simulink model "SIM_SAD_DEMO"  (R2025b)
settings: Solver=ode5  StartTime=0.0  StopTime=T/10  FixedStep=0.1  RelTol=1e-3
model workspace (MAT data in the model file):
  Pnull = Simulink.Parameter
  Pnull.Value = Simulink.data.Expression
  Pnull.Value.ExpressionString = "zeros(3,1)"
  Pnull.Complexity = 'real'
  Pnull.Dimensions = -1
  Pnull.DataType = 'auto'
  rho_albedo_medio = Simulink.Parameter
  rho_albedo_medio.Value = 0.3
  rho_albedo_medio.Complexity = 'real'
  rho_albedo_medio.Dimensions = [1 1]
  rho_albedo_medio.DataType = 'auto'
values from neighbouring files (symbols this model uses):
  Aree = zeros(10,1)    [SCRIPT_SAD_DEMO.m]    (also in lab_7.m)
  c = astroConstants(5)*1e3    [SCRIPT_SAD_DEMO.m]    (also in lab_7.m)
  draan = 1.99096871e-7    (= 1.99096871e-07)    [SCRIPT_SAD_DEMO.m]
  eps_E = deg2rad(astroConstants(63))    [SCRIPT_SAD_DEMO.m]    (also in lab_7.m)
  F_e = 1358    [SCRIPT_SAD_DEMO.m]    (also in lab_7.m)
  j_B = [0.01; 0.05; 0.01]    [SCRIPT_SAD_DEMO.m]    (also in lab_7.m)
  J_depl = [100.9, 0, 0;           0, 25.1, 0;           0, 0, 91.6]*1e-2    [SCRIPT_SAD_DEMO.m]    (also in lab_7.m)
  JD0 = juliandate(startTime)    [SCRIPT_SAD_DEMO.m]
  kep = [a,e,incl,raan,w,theta]    [SCRIPT_SAD_DEMO.m]    (also in lab_7.m)
  mu = astroConstants(13)    [SCRIPT_SAD_DEMO.m]    (also in lab_7.m)
  n = sqrt( (mu/ (a)^3))    [SCRIPT_SAD_DEMO.m]    (also in lab_7.m = sqrt((mu/ ((a/1000)^3))))
  n_sun = 2*pi/T_sun    (= 1.99238499086e-07)    [SCRIPT_SAD_DEMO.m]    (also in lab_7.m)
  Nmat = [ ... (first row only)    [SCRIPT_SAD_DEMO.m]    (also in lab_7.m)
  r_sun = 1*AU    [SCRIPT_SAD_DEMO.m]    (also in lab_7.m = 1*ua)
  Re = astroConstants(23)    [SCRIPT_SAD_DEMO.m]    (also in lab_7.m)
  rf = [ ... (first row only)    [SCRIPT_SAD_DEMO.m]    (also in lab_7.m)
  rhod = 0.1*ones(10,1)    [SCRIPT_SAD_DEMO.m]    (also in lab_7.m)
  rhos = zeros(10,1)    [SCRIPT_SAD_DEMO.m]    (also in lab_7.m)
  theta = 0    [SCRIPT_SAD_DEMO.m]    (also in lab_7.m)
undefined symbols (not defined in the file or in its folder): avec, bvec, DiscIntNeverNeededParam, dspblkCoreblockFVToolHelper, gcbh, Gyro, Magmeter, q, SRP, Sun_sensor
libraries: LIBRARY_SAD x37, matrix_library x28
(part 1 of 3)
settings Model: Creator=fabio  LastModifiedBy=delil

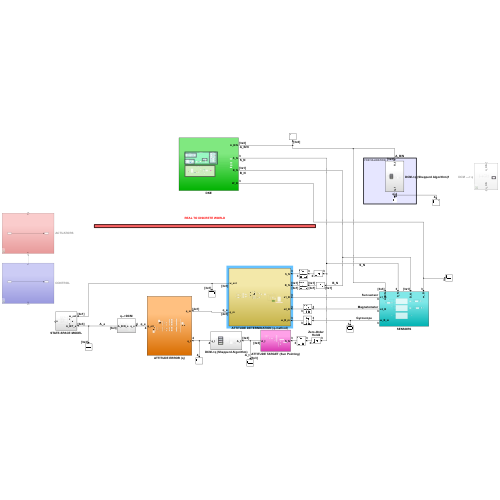
[thumbnail: Simulink's stored preview of the top-level diagram]
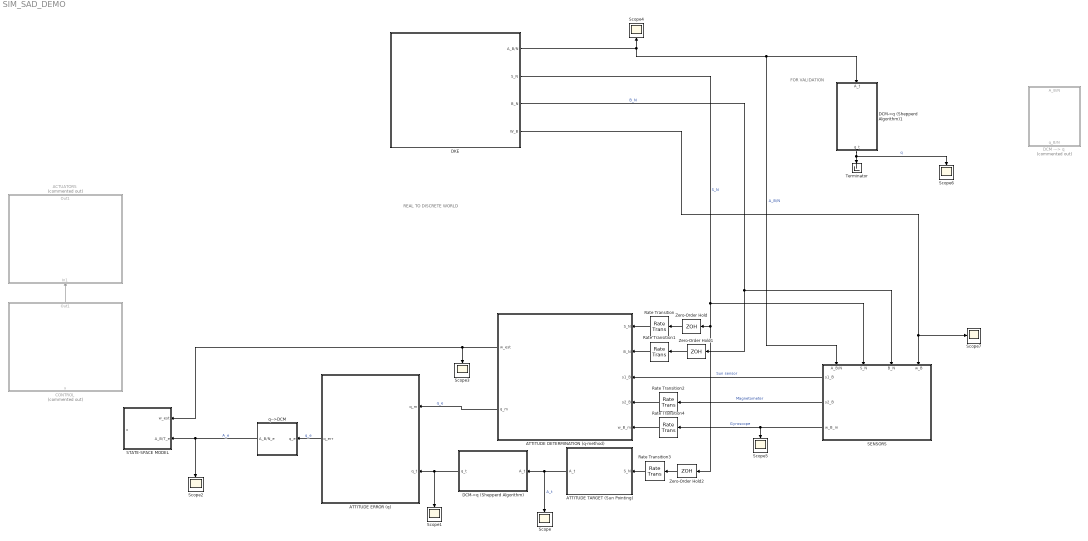
== system SIM_SAD_DEMO ==
  note: FOR VALIDATION
  note: REAL TO DISCRETE WORLD
  ACTUATORS : Subsystem  Commented=on
  ATTITUDE DETERMINATION (q-method) : Subsystem
  ATTITUDE ERROR (q) : Subsystem
  ATTITUDE TARGET (Sun Pointing) : Subsystem
  CONTROL : Subsystem  Commented=on
  DCM ---> q : Subsystem  Commented=on
  DCM->q (Shepperd Algorithm) : Subsystem
  DCM->q (Shepperd Algorithm)1 : Subsystem
  DKE : Subsystem
  Rate Transition{,1..4} (5 alike) : RateTransition  OutPortSampleTime=max(Sun_sensor.Ts,Magmeter.Ts)
  SENSORS : Subsystem
      settings: PortSchema="{\"entries\":[{\"content\":{\"sides\":[{\"content\":{\"connectorIds\":[\"In1\",\"In2\",\"In3\",\"In4\"]},\"type\":\"ConnectorPlacement.EquallySpacedRectSide\",\"uuid\":\"40962b30-3bcb-49e0-bc68-6aa3a31cfc97\"},{\"content\":{\"side\":\"RIGHT\"},\"type\":\"ConnectorPlacement.EquallySpacedRectSide\",\"uuid\":\"a8221d80-3d13-495d-884e-34f2ccc75f25\"},{\"content\":{\"connectorIds\":[\"Out1\",\"Out2\",\"Out3\"],\"side\":\"TOP\"},\"type\":\"ConnectorPlacement.EquallySpacedRectSide\",\"uuid\":\"62b0f620-b15f-4d6a-bcfa-939a48d36217\"}]},\"type\":\"ConnectorPlacement.EquallySpacedConnector\",\"uuid\":\"bc93d320-282b-4258-8528-17688a47c52b\"}],\"packageUris\":[\"http://schema.mathworks.com/mf0/Connector/R2020b\"],\"version\":\"1.0\"}"
  STATE-SPACE MODEL : Subsystem
  Scope{,1..7} (8 alike) : Scope
      Scope settings: ActiveDisplayYMinimum=-1  ActiveDisplayYMaximum=1  DataLoggingVariableName=ScopeData55
      Scope1 settings: ActiveDisplayYMinimum=-1  ActiveDisplayYMaximum=1  DataLoggingVariableName=ScopeData81
      Scope2 settings: ActiveDisplayYMinimum=-1.2400140928314325  ActiveDisplayYMaximum=1.248890454759048  DataLoggingVariableName=ScopeData60
      Scope3 settings: ActiveDisplayYMinimum=-0.92000036614875291  ActiveDisplayYMaximum=5.28182468939155  DataLoggingVariableName=ScopeData72
      Scope4 settings: ActiveDisplayYMinimum=-1.2499999997091158  ActiveDisplayYMaximum=1.2499999999676794  DataLoggingVariableName=ScopeData71
      Scope5 settings: ActiveDisplayYMinimum=-0.010336393980870042  ActiveDisplayYMaximum=0.027780099120889055  DataLoggingVariableName=ScopeData83
      Scope6 settings: ActiveDisplayYMinimum=-1  ActiveDisplayYMaximum=1  DataLoggingVariableName=ScopeData82
      Scope7 settings: ActiveDisplayYMinimum=-0.018485878503427311  ActiveDisplayYMaximum=0.018741294883568061  DataLoggingVariableName=ScopeData84
  Terminator : Terminator
  Zero-Order Hold : ZeroOrderHold  SampleTime=max(Sun_sensor.Ts,Magmeter.Ts)
  Zero-Order Hold1 : ZeroOrderHold  SampleTime=max(Sun_sensor.Ts,Magmeter.Ts)
  Zero-Order Hold2 : ZeroOrderHold  SampleTime=max(Sun_sensor.Ts,Magmeter.Ts)
  q-->DCM : Subsystem
  wires:
  DCM->q (Shepperd Algorithm)1/1(q_t) -> Scope6/1, Terminator/1  "q"
  SENSORS/2(s2_B) -> Rate Transition2/1  "Magnetometer"
  ATTITUDE TARGET (Sun Pointing)/1(A_t) -> Scope/1, DCM->q (Shepperd Algorithm)/1(A_t)  "A_t"
  DCM->q (Shepperd Algorithm)/1(q_t) -> Scope1/1, ATTITUDE ERROR (q)/2(q_t)
  q-->DCM/1(A_B/N_e) -> Scope2/1, STATE-SPACE MODEL/2(A_B/T_e)  "A_e"
  ATTITUDE ERROR (q)/1(q_err) -> q-->DCM/1(q_e)  "q_e"
  Zero-Order Hold/1 -> Rate Transition/1
  Rate Transition/1 -> ATTITUDE DETERMINATION (q-method)/1(S_N)
  Zero-Order Hold1/1 -> Rate Transition1/1
  Rate Transition1/1 -> ATTITUDE DETERMINATION (q-method)/2(B_N)
  Zero-Order Hold2/1 -> Rate Transition3/1
  Rate Transition3/1 -> ATTITUDE TARGET (Sun Pointing)/1(S_N)
  CONTROL/1(Out1) -> ACTUATORS/1(In1)
  DKE/4(W_B) -> SENSORS/4(w_B), Scope7/1
  SENSORS/3(w_B_m) -> Scope5/1, Rate Transition4/1  "Gyroscope"
  ATTITUDE DETERMINATION (q-method)/2(q_m) -> ATTITUDE ERROR (q)/1(q_m)  "q_e"
  Rate Transition2/1 -> ATTITUDE DETERMINATION (q-method)/4(s2_B)
  ATTITUDE DETERMINATION (q-method)/1(w_est) -> Scope3/1, STATE-SPACE MODEL/1(w_est)
  DKE/3(B_N) -> SENSORS/3("B_N "), Zero-Order Hold1/1  "B_N"
  SENSORS/1(s1_B) -> ATTITUDE DETERMINATION (q-method)/3(s1_B)  "Sun sensor"
  DKE/2(S_N) -> SENSORS/2(S_N), Zero-Order Hold/1, Zero-Order Hold2/1  "S_N"
  DKE/1(A_B/N) -> Scope4/1, DCM->q (Shepperd Algorithm)1/1(A_t), SENSORS/1(A_B/N)  "A_B/N"
  Rate Transition4/1 -> ATTITUDE DETERMINATION (q-method)/5(w_B_m)

== system SIM_SAD_DEMO/ACTUATORS ==
  In1 : Inport
  Out1 : Outport
  wires:
  In1/1 -> Out1/1

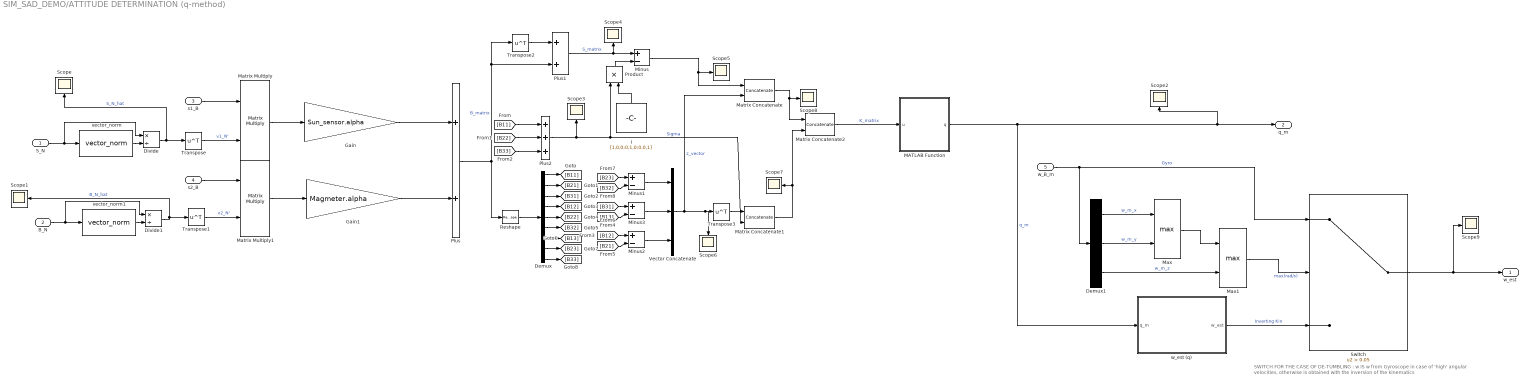
== system SIM_SAD_DEMO/ATTITUDE DETERMINATION (q-method) ==
  note: SWITCH FOR THE CASE OF DE-TUMBLING : w IS w from Gyroscope in case of 'high' angular velocities, otherwise is obtained with the inversion of the kinematics
  S_N : Inport
  B_N : Inport  Port=2
  s1_B : Inport  Port=3
  s2_B : Inport  Port=4
  w_B_m : Inport  Port=5
  Demux : Demux  Outputs=9
  Demux1 : Demux  Outputs=3
  Divide : Product  Inputs=*/
  Divide1 : Product  Inputs=*/
  Gain : Gain  Gain=Sun_sensor.alpha
  Gain1 : Gain  Gain=Magmeter.alpha
  I : Constant  Value=[1,0,0;0,1,0;0,0,1]
  MATLAB Function : MATLAB Function  TreatAsAtomicUnit=on  SystemSampleTime=q.Ts
  Matrix Concatenate : Concatenate  Mode=Multidimensional array  ConcatenateDimension=2
  Matrix Concatenate1 : Concatenate  Mode=Multidimensional array  ConcatenateDimension=2
  Matrix Concatenate2 : Concatenate  Mode=Multidimensional array
  Matrix Multiply : Product  Multiplication=Matrix(*)
  Matrix Multiply1 : Product  Multiplication=Matrix(*)
  Max : MinMax  Function=max  Inputs=2
  Max1 : MinMax  Function=max  Inputs=2
  Minus{,1..3} (4 alike) : Sum  Inputs=+-
  Plus : Sum
  Plus1 : Sum
  Plus2 : Sum  Inputs=+++
  Product : Product
  Reshape : Reshape  OutputDimensionality=Customize  OutputDimensions=[9,1]
  Scope{,1..9} (10 alike) : Scope
      Scope settings: ActiveDisplayYMinimum=-0.12499999999999997  ActiveDisplayYMaximum=1.125  DataLoggingVariableName=ScopeData61
      Scope1 settings: ActiveDisplayYMinimum=-0.60786913937993192  ActiveDisplayYMaximum=1.0990417923572595  DataLoggingVariableName=ScopeData62
      Scope2 settings: ActiveDisplayYMinimum=-0.9533532616313245  ActiveDisplayYMaximum=1.1062124291352333  DataLoggingVariableName=ScopeData74
      Scope3 settings: ActiveDisplayYMinimum=-1  ActiveDisplayYMaximum=1  DataLoggingVariableName=ScopeData75
      Scope4 settings: DataLoggingVariableName=ScopeData76
      Scope5 settings: ActiveDisplayYMinimum=-1  ActiveDisplayYMaximum=1  DataLoggingVariableName=ScopeData77
      Scope6 settings: DataLoggingVariableName=ScopeData78
      Scope7 settings: ActiveDisplayYMinimum=-1  ActiveDisplayYMaximum=1  DataLoggingVariableName=ScopeData79
      Scope8 settings: ActiveDisplayYMinimum=-1.2343387282561236  ActiveDisplayYMaximum=1.1812725103052406  DataLoggingVariableName=ScopeData80
      Scope9 settings: ActiveDisplayYMinimum=-0.28605679058813616  ActiveDisplayYMaximum=0.3787347965228936  DataLoggingVariableName=ScopeData85
  Switch : Switch  Criteria=u2 > Threshold  Threshold=0.05  SaturateOnIntegerOverflow=off  InputSameDT=off
  Transpose{,1..3} (4 alike) : Math  Operator=transpose
  Vector Concatenate : Concatenate  NumInputs=3
  vector_norm : LIBRARY_SAD/vector_norm  SystemSampleTime=-1  VariantActivationTime=update diagram  EmptyChoice=off  PassThrough=off  PassThroughVariantControl=(default)  EmptyChoiceVariantControl=(default)  AllowFlexibleInterface=on  Latency=0  AutoFrameSizeCalculation=off
  vector_norm1 : LIBRARY_SAD/vector_norm  SystemSampleTime=-1  VariantActivationTime=update diagram  EmptyChoice=off  PassThrough=off  PassThroughVariantControl=(default)  EmptyChoiceVariantControl=(default)  AllowFlexibleInterface=on  Latency=0  AutoFrameSizeCalculation=off
  w_est (q) : Subsystem
  w_est : Outport
  q_m : Outport  Port=2
  wires:
  vector_norm/1 -> Divide/2
  Demux/6 -> [B32]
  Divide/1 -> Scope/1, Transpose/1  "S_N_hat"
  Gain/1 -> Plus/1
  [B32] -> Minus1/2
  Gain1/1 -> Plus/2
  S_N/1 -> Divide/1, vector_norm/1
  Plus2/1 -> Scope3/1, Product/1, Matrix Concatenate1/2  "Sigma"
  B_N/1 -> Divide1/1, vector_norm1/1
  Demux/4 -> [B12]
  Plus/1 -> Reshape/1, Transpose2/1, Plus1/2  "B_matrix"
  Divide1/1 -> Scope1/1, Transpose1/1  "B_N_hat"
  [B12] -> Minus2/1
  Demux/3 -> [B31]
  Demux/8 -> [B23]
  Vector Concatenate/1 -> Matrix Concatenate/2, Transpose3/1, Scope6/1  "z_vector"
  Minus1/1 -> Vector Concatenate/1
  Minus2/1 -> Vector Concatenate/3
  Transpose2/1 -> Plus1/1
  [B11] -> Plus2/1
  Transpose/1 -> Matrix Multiply/2  "v1_N'"
  Minus/1 -> Scope5/1, Matrix Concatenate/1
  Matrix Concatenate1/1 -> Scope7/1, Matrix Concatenate2/2
  Demux/1 -> [B11]
  [B22] -> Plus2/2
  Matrix Multiply1/1 -> Gain1/1
  Demux/2 -> [B21]
  [B23] -> Minus1/1
  Demux/5 -> [B22]
  Matrix Multiply/1 -> Gain/1
  Demux/9 -> [B33]
  Reshape/1 -> Demux/1
  Demux/7 -> [B13]
  vector_norm1/1 -> Divide1/2
  [B33] -> Plus2/3
  Matrix Concatenate/1 -> Matrix Concatenate2/1, Scope8/1
  Transpose1/1 -> Matrix Multiply1/2  "v2_N'"
  Transpose3/1 -> Matrix Concatenate1/1
  Minus3/1 -> Vector Concatenate/2
  [B31] -> Minus3/1
  Plus1/1 -> Minus/1, Scope4/1  "S_matrix"
  [B13] -> Minus3/2
  [B21] -> Minus2/2
  Product/1 -> Minus/2
  I/1 -> Product/2
  s1_B/1 -> Matrix Multiply/1
  s2_B/1 -> Matrix Multiply1/1
  MATLAB Function/1(q) -> w_est (q)/1(q_m), q_m/1, Scope2/1  "q_m"
  Switch/1 -> Scope9/1, w_est/1
  Matrix Concatenate2/1 -> MATLAB Function/1(u)  "K_matrix"
  Max/1 -> Max1/1
  Demux1/3 -> Max1/2  "w_m_z"
  Demux1/2 -> Max/2  "w_m_y"
  Demux1/1 -> Max/1  "w_m_x"
  w_B_m/1 -> Switch/1, Demux1/1  "Gyro"
  Max1/1 -> Switch/2  "max(rad/s)"
  w_est (q)/1(w_est) -> Switch/3  "Inverting Kin"

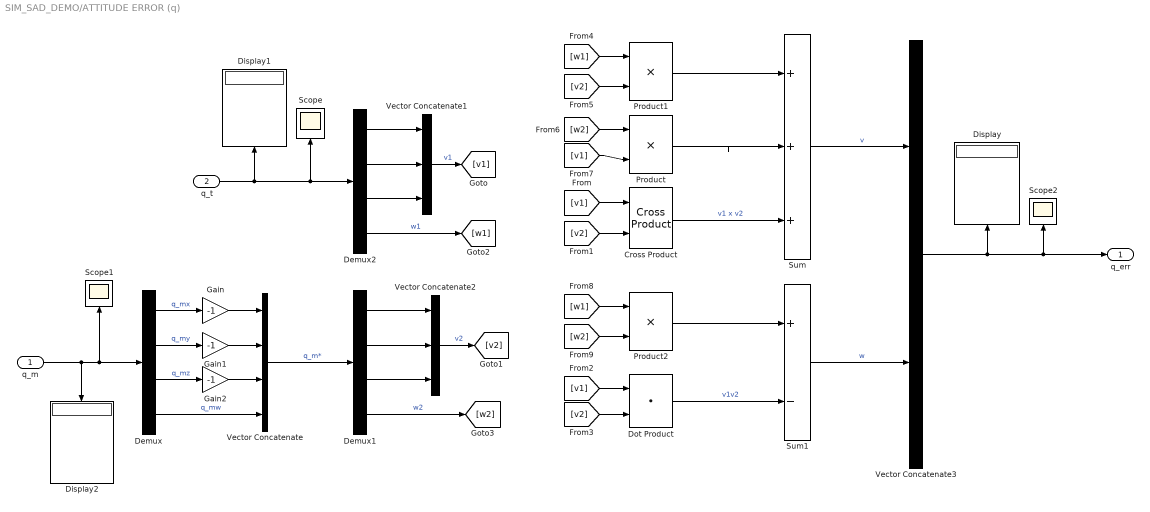
== system SIM_SAD_DEMO/ATTITUDE ERROR (q) ==
  q_m : Inport
  q_t : Inport  Port=2
  Cross Product : matrix_library/Cross Product
  Demux : Demux
  Demux1 : Demux
  Demux2 : Demux
  Display : Display
  Display1 : Display
  Display2 : Display
  Dot Product : DotProduct  OutDataTypeStr=Inherit: Inherit via internal rule
  Gain : Gain  Gain=-1
  Gain1 : Gain  Gain=-1
  Gain2 : Gain  Gain=-1
  Product : Product
  Product1 : Product
  Product2 : Product
  Scope : Scope
      settings: ActiveDisplayYMinimum=-0.12923710595911297  ActiveDisplayYMaximum=1.1085905151201327  DataLoggingVariableName=ScopeData63
  Scope1 : Scope
      settings: ActiveDisplayYMinimum=-1.1944830769885011  ActiveDisplayYMaximum=1.2235445279118087  DataLoggingVariableName=ScopeData64
  Scope2 : Scope
      settings: ActiveDisplayYMinimum=-1  ActiveDisplayYMaximum=1  DataLoggingVariableName=ScopeData65
  Sum : Sum  Inputs=+++
  Sum1 : Sum  Inputs=+-
  Vector Concatenate : Concatenate  NumInputs=4
  Vector Concatenate1 : Concatenate  NumInputs=3
  Vector Concatenate2 : Concatenate  NumInputs=3
  Vector Concatenate3 : Concatenate
  q_err : Outport
  wires:
  q_m/1 -> Scope1/1, Demux/1, Display2/1
  q_t/1 -> Demux2/1, Scope/1, Display1/1
  Demux/1 -> Gain/1  "q_mx"
  Demux/2 -> Gain1/1  "q_my"
  Demux/3 -> Gain2/1  "q_mz"
  Demux/4 -> Vector Concatenate/4  "q_mw"
  Gain2/1 -> Vector Concatenate/3
  Gain1/1 -> Vector Concatenate/2
  Gain/1 -> Vector Concatenate/1
  Vector Concatenate/1 -> Demux1/1  "q_m*"
  Demux1/1 -> Vector Concatenate2/1
  Demux1/2 -> Vector Concatenate2/2
  Demux1/3 -> Vector Concatenate2/3
  Demux1/4 -> [w2]  "w2"
  Demux2/1 -> Vector Concatenate1/1
  Demux2/2 -> Vector Concatenate1/2
  Demux2/3 -> Vector Concatenate1/3
  Vector Concatenate1/1 -> [v1]  "v1"
  Demux2/4 -> [w1]  "w1"
  Cross Product/1 -> Sum/3  "v1 x v2"
  Dot Product/1 -> Sum1/2  "v1v2"
  [v1] -> Cross Product/1
  Vector Concatenate2/1 -> [v2]  "v2"
  [v2] -> Cross Product/2
  [v1] -> Dot Product/1
  [v2] -> Dot Product/2
  [w1] -> Product1/1
  [v2] -> Product1/2
  [v1] -> Product/2
  [w2] -> Product/1
  Product1/1 -> Sum/1
  Product/1 -> Sum/2
  [w1] -> Product2/1
  [w2] -> Product2/2
  Product2/1 -> Sum1/1
  Sum/1 -> Vector Concatenate3/1  "v"
  Sum1/1 -> Vector Concatenate3/2  "w"
  Vector Concatenate3/1 -> Scope2/1, q_err/1, Display/1

== system SIM_SAD_DEMO/ATTITUDE TARGET (Sun Pointing) ==
  note: BORESIGHT AXIS : axis which points the Sun
  S_N : Inport
  Constant{1..2,4,6,8..11} (8 alike) : Constant  Value=0
  Constant{3,5,7,12} (4 alike) : Constant
  Cross Product : matrix_library/Cross Product
  Cross Product1 : matrix_library/Cross Product
  Display : Display
  Display1 : Display
  MatrixMultiply : Product  Multiplication=Matrix(*)
  Normalized Vector : Subsystem
  Normalized Vector2 : Subsystem
  Scope{,1..4} (5 alike) : Scope
      Scope settings: ActiveDisplayYMinimum=-1  ActiveDisplayYMaximum=1  DataLoggingVariableName=ScopeData62
      Scope1 settings: ActiveDisplayYMinimum=-1  ActiveDisplayYMaximum=1  DataLoggingVariableName=ScopeData66
      Scope2 settings: ActiveDisplayYMinimum=-1  ActiveDisplayYMaximum=1  DataLoggingVariableName=ScopeData69
      Scope3 settings: ActiveDisplayYMinimum=-1  ActiveDisplayYMaximum=1  DataLoggingVariableName=ScopeData70
      Scope4 settings: ActiveDisplayYMinimum=-1  ActiveDisplayYMaximum=1  DataLoggingVariableName=ScopeData73
  Sum : Sum  Inputs=|+-
  Transpose : Math  Operator=transpose
  Vector Concatenate : Concatenate  NumInputs=3  Mode=Multidimensional array  ConcatenateDimension=2
  Vector Concatenate{1..4} (4 alike) : Concatenate  NumInputs=3
  Vector Concatenate5 : Concatenate  NumInputs=3  Mode=Multidimensional array  ConcatenateDimension=2
  A_t : Outport
  wires:
  S_N/1 -> Normalized Vector2/1(r)
  Normalized Vector2/1(s2_B) -> Cross Product/2, Cross Product1/1, Scope/1, Vector Concatenate/1  "x_t_hat"
  Vector Concatenate1/1 -> Cross Product/1  "k_hat"
  Cross Product/1 -> Normalized Vector/1(In1)
  Normalized Vector/1(Out1) -> Scope1/1, Vector Concatenate/2, Cross Product1/2  "y_t_hat"
  Cross Product1/1 -> Scope2/1, Vector Concatenate/3  "z_t_hat"
  Vector Concatenate/1 -> Scope4/1, A_t/1, MatrixMultiply/2, Transpose/1, Display/1  "A_T/N"
  Transpose/1 -> MatrixMultiply/1
  MatrixMultiply/1 -> Sum/1
  Vector Concatenate5/1 -> Display1/1, Sum/2  "I_matrix"
  Sum/1 -> Scope3/1
  Constant2/1 -> Vector Concatenate1/2
  Constant1/1 -> Vector Concatenate1/1
  Constant3/1 -> Vector Concatenate1/3
  Constant6/1 -> Vector Concatenate2/3
  Constant4/1 -> Vector Concatenate2/1
  Constant5/1 -> Vector Concatenate2/2
  Constant8/1 -> Vector Concatenate3/2
  Constant7/1 -> Vector Concatenate3/1
  Constant9/1 -> Vector Concatenate3/3
  Constant11/1 -> Vector Concatenate4/2
  Constant10/1 -> Vector Concatenate4/1
  Constant12/1 -> Vector Concatenate4/3
  Vector Concatenate3/1 -> Vector Concatenate5/1
  Vector Concatenate2/1 -> Vector Concatenate5/2
  Vector Concatenate4/1 -> Vector Concatenate5/3

== system SIM_SAD_DEMO/CONTROL ==
  x : Inport
  Out1 : Outport
  wires:
  x/1 -> Out1/1

== system SIM_SAD_DEMO/DCM ---> q ==
  note: CHECK BY RECONSTRUCTING A_B/N AND ORTHONORMALITY ERROR
  A_B/N : Inport
  Constant : Constant
  Demux : Demux  Outputs=9
  Divide{,1..3} (4 alike) : Product  Inputs=*/
  Gain : Gain  Gain=4
  Gain1 : Gain  Gain=4
  Gain2 : Gain  Gain=4
  Gain3 : Gain  Gain=1/2
  Reshape : Reshape  OutputDimensionality=Customize  OutputDimensions=[9,1]
  Sqrt : Sqrt
  Sum : Sum  Inputs=+-
  Sum1 : Sum  Inputs=++++
  Sum2 : Sum  Inputs=+-
  Sum3 : Sum  Inputs=+-
  Transpose1 : Math  Operator=transpose
  Vector Concatenate : Concatenate  NumInputs=4
  q-->DCM (CHECK) : Subsystem  Commented=on
  vector_norm : Subsystem
  q_B/N : Outport
  wires:
  A_B/N/1 -> Transpose1/1  "A_B/N"
  Transpose1/1 -> Reshape/1
  Divide3/1 -> q_B/N/1, q-->DCM (CHECK)/1(q_norm)  "q_norm"
  vector_norm/1(r_norm) -> Divide3/2
  Gain3/1 -> Vector Concatenate/4, Gain/1, Gain2/1, Gain1/1  "q4"
  Sqrt/1 -> Gain3/1
  Vector Concatenate/1 -> vector_norm/1(r), Divide3/1  "q"
  Gain2/1 -> Divide2/2
  Sum3/1 -> Divide2/1
  Gain1/1 -> Divide1/2
  Sum2/1 -> Divide1/1
  Gain/1 -> Divide/2
  Sum/1 -> Divide/1
  Constant/1 -> Sum1/1
  Sum1/1 -> Sqrt/1
  Divide2/1 -> Vector Concatenate/3  "q3"
  Divide1/1 -> Vector Concatenate/2  "q2"
  Divide/1 -> Vector Concatenate/1  "q1"
  Demux/9 -> Sum1/4  "A_33"
  Demux/8 -> Sum/2  "A_32"
  Demux/7 -> Sum2/1  "A_31"
  Demux/6 -> Sum/1  "A_23"
  Demux/5 -> Sum1/3  "A_22"
  Demux/4 -> Sum3/2  "A_21"
  Demux/3 -> Sum2/2  "A_13"
  Demux/2 -> Sum3/1  "A_12"
  Demux/1 -> Sum1/2  "A_11"
  Reshape/1 -> Demux/1

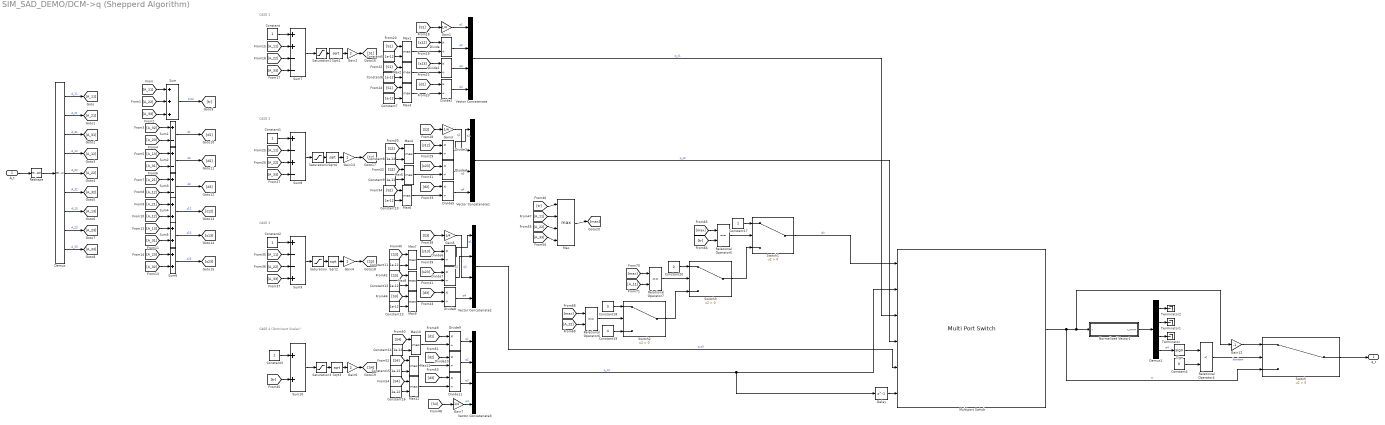
== system SIM_SAD_DEMO/DCM->q (Shepperd Algorithm) ==
  note: CASE 1
  note: CASE 2
  note: CASE 3
  note: CASE 4 (Dominant Scalar)
  A_t : Inport
  Constant{,1..3,17} (5 alike) : Constant
  Constant{5..16} (12 alike) : Constant  Value=1e-12
  Constant18 : Constant  Value=3
  Constant19 : Constant  Value=4
  Constant20 : Constant  Value=2
  Constant4 : Constant  Value=0
  Delay : Delay  DelayLength=1
  Demux : Demux  Outputs=9
  Demux1 : Demux
  Divide{,1..11} (12 alike) : Product  Inputs=*/
  Gain{1,3,5,7} (4 alike) : Gain  Gain=1/4
  Gain12 : Gain  Gain=-1
  Gain{2,4,6,13} (4 alike) : Gain  Gain=2
  Max : MinMax  Function=max  Inputs=4
  Max{1..12} (12 alike) : MinMax  Function=max  Inputs=2
  Multiport Switch : MultiPortSwitch  Inputs=4  DataPortForDefault=Additional data port  DiagnosticForDefault=Warning  SaturateOnIntegerOverflow=off
  Normalized Vector1 : Subsystem
  Relational Operator4 : RelationalOperator  Operator=<  OutDataTypeStr=boolean  RndMeth=Simplest  InputSameDT=off
  Relational Operator5 : RelationalOperator  Operator===  OutDataTypeStr=boolean  RndMeth=Simplest  InputSameDT=off
  Relational Operator6 : RelationalOperator  Operator===  OutDataTypeStr=boolean  RndMeth=Simplest  InputSameDT=off
  Relational Operator7 : RelationalOperator  Operator===  OutDataTypeStr=boolean  RndMeth=Simplest  InputSameDT=off
  Reshape : Reshape  OutputDimensionality=Customize  OutputDimensions=[9,1]
  Saturation{,1..3} (4 alike) : Saturate  UpperLimit=inf  LowerLimit=0
  Sign : Signum
  Sqrt{1..4} (4 alike) : Sqrt
  Sum : Sum  Inputs=+++
  Sum1 : Sum  Inputs=+-
  Sum{4..6,10} (4 alike) : Sum
  Sum2 : Sum  Inputs=+-
  Sum3 : Sum  Inputs=+-
  Sum7 : Sum  Inputs=++--
  Sum8 : Sum  Inputs=+-+-
  Sum9 : Sum  Inputs=+--+
  Switch{,1..3} (4 alike) : Switch  Criteria=u2 > Threshold  SaturateOnIntegerOverflow=off  InputSameDT=off
  Terminator : Terminator
  Terminator1 : Terminator
  Terminator2 : Terminator
  Vector Concatenate{,1..3} (4 alike) : Concatenate  NumInputs=4
  q_t : Outport
  wires:
  A_t/1 -> Reshape/1
  Reshape/1 -> Demux/1
  Demux/1 -> [A_11]  "A_11"
  Demux/2 -> [A_21]  "A_21"
  Demux/3 -> [A_31]  "A_31"
  Demux/4 -> [A_12]  "A_12"
  Demux/5 -> [A_22]  "A_22"
  Demux/6 -> [A_32]  "A_32"
  Demux/7 -> [A_13]  "A_13"
  Demux/8 -> [A_23]  "A_23"
  Demux/9 -> [A_33]  "A_33"
  Sum/1 -> [tr]  "tr(A)"
  [A_11] -> Sum/1
  [A_22] -> Sum/2
  [A_33] -> Sum/3
  [A_32] -> Sum1/1
  [A_23] -> Sum1/2
  Sum1/1 -> [d1]  "d1"
  Sum2/1 -> [d2]  "d2"
  [A_31] -> Sum2/2
  [A_13] -> Sum2/1
  [A_21] -> Sum3/1
  [A_12] -> Sum3/2
  Sum3/1 -> [d3]  "d3"
  Sum4/1 -> [s12]  "s12"
  [A_12] -> Sum4/2
  [A_21] -> Sum4/1
  [A_13] -> Sum5/1
  [A_31] -> Sum5/2
  Sum5/1 -> [s13]  "s13"
  Sum6/1 -> [s23]  "s23"
  [A_32] -> Sum6/2
  [A_23] -> Sum6/1
  [A_11] -> Sum7/2
  [A_22] -> Sum7/3
  [A_33] -> Sum7/4
  Constant/1 -> Sum7/1
  Sum7/1 -> Saturation2/1
  Gain2/1 -> [S1]
  [S1] -> Gain1/1
  Gain1/1 -> Vector Concatenate/1  "q1"
  [s12] -> Divide/1
  Divide/1 -> Vector Concatenate/2  "q2"
  Divide1/1 -> Vector Concatenate/3  "q3"
  [s13] -> Divide1/1
  [d1] -> Divide2/1
  Divide2/1 -> Vector Concatenate/4  "q4"
  Vector Concatenate/1 -> Multiport Switch/3  "q_c1"
  Vector Concatenate1/1 -> Multiport Switch/4  "q_c2"
  Divide5/1 -> Vector Concatenate1/4  "q4"
  [d2] -> Divide5/1
  [s23] -> Divide4/1
  Divide4/1 -> Vector Concatenate1/3  "q3"
  Divide3/1 -> Vector Concatenate1/1  "q1"
  [s12] -> Divide3/1
  Gain3/1 -> Vector Concatenate1/2  "q2"
  [S2] -> Gain3/1
  Gain13/1 -> [S2]
  Sum8/1 -> Saturation1/1
  Constant1/1 -> Sum8/1
  [A_33] -> Sum8/4
  [A_22] -> Sum8/3
  [A_11] -> Sum8/2
  [A_11] -> Sum9/2
  [A_22] -> Sum9/3
  [A_33] -> Sum9/4
  Constant2/1 -> Sum9/1
  Sum9/1 -> Saturation/1
  Sqrt2/1 -> Gain4/1
  Gain4/1 -> [S3]
  [S3] -> Gain5/1
  Gain5/1 -> Vector Concatenate2/3  "q3"
  [s13] -> Divide6/1
  Divide6/1 -> Vector Concatenate2/1  "q1"
  Divide7/1 -> Vector Concatenate2/2  "q2"
  Max8/1 -> Divide7/2
  [s23] -> Divide7/1
  [d3] -> Divide8/1
  Max9/1 -> Divide8/2
  Divide8/1 -> Vector Concatenate2/4  "q4"
  Vector Concatenate2/1 -> Multiport Switch/5  "q_c3"
  Vector Concatenate3/1 -> Multiport Switch/2, Delay/1  "q_c4"
  Divide11/1 -> Vector Concatenate3/3  "q3"
  [d3] -> Divide11/1
  [d2] -> Divide10/1
  Divide10/1 -> Vector Concatenate3/2  "q2"
  Divide9/1 -> Vector Concatenate3/1  "q1"
  [d1] -> Divide9/1
  Gain7/1 -> Vector Concatenate3/4  "q4"
  [S4] -> Gain7/1
  Gain6/1 -> [S4]
  Constant3/1 -> Sum10/1
  [tr] -> Sum10/2
  [tr] -> Max/1
  [A_11] -> Max/2
  [A_22] -> Max/3
  [A_33] -> Max/4
  Max/1 -> [max]
  Delay/1 -> Multiport Switch/6
  Multiport Switch/1 -> Switch/3, Gain12/1, Normalized Vector1/1(r)  "q"
  Normalized Vector1/1(r_norm) -> Demux1/1
  Demux1/4 -> Sign/1  "q4"
  Sign/1 -> Relational Operator4/1
  Demux1/3 -> Terminator/1
  Demux1/2 -> Terminator1/1
  Demux1/1 -> Terminator2/1
  Constant4/1 -> Relational Operator4/2
  Relational Operator4/1 -> Switch/2  "boolean"
  Gain12/1 -> Switch/1
  Switch/1 -> q_t/1
  Saturation/1 -> Sqrt2/1
  Saturation1/1 -> Sqrt4/1
  Sqrt4/1 -> Gain13/1
  Sqrt1/1 -> Gain2/1
  Saturation2/1 -> Sqrt1/1
  Saturation3/1 -> Sqrt3/1
  Sqrt3/1 -> Gain6/1
  Sum10/1 -> Saturation3/1
  [S1] -> Max1/1
  Constant5/1 -> Max1/2
  Max1/1 -> Divide/2
  Max2/1 -> Divide1/2
  Constant6/1 -> Max2/2
  [S1] -> Max2/1
  [S1] -> Max3/1
  Constant7/1 -> Max3/2
  Max3/1 -> Divide2/2
  [S2] -> Max4/1
  Constant8/1 -> Max4/2
  Max4/1 -> Divide3/2
  Max5/1 -> Divide4/2
  Constant9/1 -> Max5/2
  [S2] -> Max5/1
  [S2] -> Max6/1
  Constant10/1 -> Max6/2
  Max6/1 -> Divide5/2
  [S3] -> Max7/1
  Constant11/1 -> Max7/2
  Max7/1 -> Divide6/2
  Constant12/1 -> Max8/2
  [S3] -> Max8/1
  [S3] -> Max9/1
  Constant13/1 -> Max9/2
  Constant14/1 -> Max10/2
  [S4] -> Max10/1
  Max10/1 -> Divide9/2
  [S4] -> Max11/1
  Constant15/1 -> Max11/2
  Max11/1 -> Divide10/2
  Constant16/1 -> Max12/2
  [S4] -> Max12/1
  Max12/1 -> Divide11/2
  Relational Operator5/1 -> Switch1/2
  [tr] -> Relational Operator5/2
  [max] -> Relational Operator5/1
  Constant17/1 -> Switch1/1
  Switch3/1 -> Switch1/3
  Switch1/1 -> Multiport Switch/1  "idx"
  Constant18/1 -> Switch2/1
  Constant19/1 -> Switch2/3
  [max] -> Relational Operator6/1
  [A_22] -> Relational Operator6/2
  Relational Operator6/1 -> Switch2/2
  Relational Operator7/1 -> Switch3/2
  [A_11] -> Relational Operator7/2
  [max] -> Relational Operator7/1
  Constant20/1 -> Switch3/1
  Switch2/1 -> Switch3/3

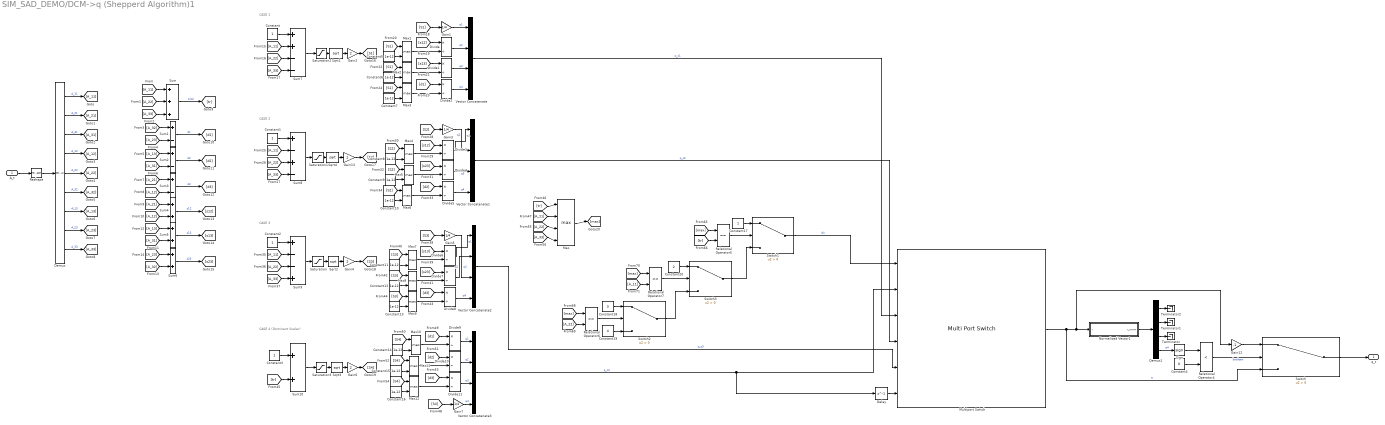
== system SIM_SAD_DEMO/DCM->q (Shepperd Algorithm)1 ==
  note: CASE 1
  note: CASE 2
  note: CASE 3
  note: CASE 4 (Dominant Scalar)
  A_t : Inport
  Constant{,1..3,17} (5 alike) : Constant
  Constant{5..16} (12 alike) : Constant  Value=1e-12
  Constant18 : Constant  Value=3
  Constant19 : Constant  Value=4
  Constant20 : Constant  Value=2
  Constant4 : Constant  Value=0
  Delay : Delay  DelayLength=1
  Demux : Demux  Outputs=9
  Demux1 : Demux
  Divide{,1..11} (12 alike) : Product  Inputs=*/
  Gain{1,3,5,7} (4 alike) : Gain  Gain=1/4
  Gain12 : Gain  Gain=-1
  Gain{2,4,6,13} (4 alike) : Gain  Gain=2
  Max : MinMax  Function=max  Inputs=4
  Max{1..12} (12 alike) : MinMax  Function=max  Inputs=2
  Multiport Switch : MultiPortSwitch  Inputs=4  DataPortForDefault=Additional data port  DiagnosticForDefault=Warning  SaturateOnIntegerOverflow=off
  Normalized Vector1 : Subsystem
  Relational Operator4 : RelationalOperator  Operator=<  OutDataTypeStr=boolean  RndMeth=Simplest  InputSameDT=off
  Relational Operator5 : RelationalOperator  Operator===  OutDataTypeStr=boolean  RndMeth=Simplest  InputSameDT=off
  Relational Operator6 : RelationalOperator  Operator===  OutDataTypeStr=boolean  RndMeth=Simplest  InputSameDT=off
  Relational Operator7 : RelationalOperator  Operator===  OutDataTypeStr=boolean  RndMeth=Simplest  InputSameDT=off
  Reshape : Reshape  OutputDimensionality=Customize  OutputDimensions=[9,1]
  Saturation{,1..3} (4 alike) : Saturate  UpperLimit=inf  LowerLimit=0
  Sign : Signum
  Sqrt{1..4} (4 alike) : Sqrt
  Sum : Sum  Inputs=+++
  Sum1 : Sum  Inputs=+-
  Sum{4..6,10} (4 alike) : Sum
  Sum2 : Sum  Inputs=+-
  Sum3 : Sum  Inputs=+-
  Sum7 : Sum  Inputs=++--
  Sum8 : Sum  Inputs=+-+-
  Sum9 : Sum  Inputs=+--+
  Switch{,1..3} (4 alike) : Switch  Criteria=u2 > Threshold  SaturateOnIntegerOverflow=off  InputSameDT=off
  Terminator : Terminator
  Terminator1 : Terminator
  Terminator2 : Terminator
  Vector Concatenate{,1..3} (4 alike) : Concatenate  NumInputs=4
  q_t : Outport
  wires:
  A_t/1 -> Reshape/1
  Reshape/1 -> Demux/1
  Demux/1 -> [A_11]  "A_11"
  Demux/2 -> [A_21]  "A_21"
  Demux/3 -> [A_31]  "A_31"
  Demux/4 -> [A_12]  "A_12"
  Demux/5 -> [A_22]  "A_22"
  Demux/6 -> [A_32]  "A_32"
  Demux/7 -> [A_13]  "A_13"
  Demux/8 -> [A_23]  "A_23"
  Demux/9 -> [A_33]  "A_33"
  Sum/1 -> [tr]  "tr(A)"
  [A_11] -> Sum/1
  [A_22] -> Sum/2
  [A_33] -> Sum/3
  [A_32] -> Sum1/1
  [A_23] -> Sum1/2
  Sum1/1 -> [d1]  "d1"
  Sum2/1 -> [d2]  "d2"
  [A_31] -> Sum2/2
  [A_13] -> Sum2/1
  [A_21] -> Sum3/1
  [A_12] -> Sum3/2
  Sum3/1 -> [d3]  "d3"
  Sum4/1 -> [s12]  "s12"
  [A_12] -> Sum4/2
  [A_21] -> Sum4/1
  [A_13] -> Sum5/1
  [A_31] -> Sum5/2
  Sum5/1 -> [s13]  "s13"
  Sum6/1 -> [s23]  "s23"
  [A_32] -> Sum6/2
  [A_23] -> Sum6/1
  [A_11] -> Sum7/2
  [A_22] -> Sum7/3
  [A_33] -> Sum7/4
  Constant/1 -> Sum7/1
  Sum7/1 -> Saturation2/1
  Gain2/1 -> [S1]
  [S1] -> Gain1/1
  Gain1/1 -> Vector Concatenate/1  "q1"
  [s12] -> Divide/1
  Divide/1 -> Vector Concatenate/2  "q2"
  Divide1/1 -> Vector Concatenate/3  "q3"
  [s13] -> Divide1/1
  [d1] -> Divide2/1
  Divide2/1 -> Vector Concatenate/4  "q4"
  Vector Concatenate/1 -> Multiport Switch/3  "q_c1"
  Vector Concatenate1/1 -> Multiport Switch/4  "q_c2"
  Divide5/1 -> Vector Concatenate1/4  "q4"
  [d2] -> Divide5/1
  [s23] -> Divide4/1
  Divide4/1 -> Vector Concatenate1/3  "q3"
  Divide3/1 -> Vector Concatenate1/1  "q1"
  [s12] -> Divide3/1
  Gain3/1 -> Vector Concatenate1/2  "q2"
  [S2] -> Gain3/1
  Gain13/1 -> [S2]
  Sum8/1 -> Saturation1/1
  Constant1/1 -> Sum8/1
  [A_33] -> Sum8/4
  [A_22] -> Sum8/3
  [A_11] -> Sum8/2
  [A_11] -> Sum9/2
  [A_22] -> Sum9/3
  [A_33] -> Sum9/4
  Constant2/1 -> Sum9/1
  Sum9/1 -> Saturation/1
  Sqrt2/1 -> Gain4/1
  Gain4/1 -> [S3]
  [S3] -> Gain5/1
  Gain5/1 -> Vector Concatenate2/3  "q3"
  [s13] -> Divide6/1
  Divide6/1 -> Vector Concatenate2/1  "q1"
  Divide7/1 -> Vector Concatenate2/2  "q2"
  Max8/1 -> Divide7/2
  [s23] -> Divide7/1
  [d3] -> Divide8/1
  Max9/1 -> Divide8/2
  Divide8/1 -> Vector Concatenate2/4  "q4"
  Vector Concatenate2/1 -> Multiport Switch/5  "q_c3"
  Vector Concatenate3/1 -> Multiport Switch/2, Delay/1  "q_c4"
  Divide11/1 -> Vector Concatenate3/3  "q3"
  [d3] -> Divide11/1
  [d2] -> Divide10/1
  Divide10/1 -> Vector Concatenate3/2  "q2"
  Divide9/1 -> Vector Concatenate3/1  "q1"
  [d1] -> Divide9/1
  Gain7/1 -> Vector Concatenate3/4  "q4"
  [S4] -> Gain7/1
  Gain6/1 -> [S4]
  Constant3/1 -> Sum10/1
  [tr] -> Sum10/2
  [tr] -> Max/1
  [A_11] -> Max/2
  [A_22] -> Max/3
  [A_33] -> Max/4
  Max/1 -> [max]
  Delay/1 -> Multiport Switch/6
  Multiport Switch/1 -> Switch/3, Gain12/1, Normalized Vector1/1(r)  "q"
  Normalized Vector1/1(r_norm) -> Demux1/1
  Demux1/4 -> Sign/1  "q4"
  Sign/1 -> Relational Operator4/1
  Demux1/3 -> Terminator/1
  Demux1/2 -> Terminator1/1
  Demux1/1 -> Terminator2/1
  Constant4/1 -> Relational Operator4/2
  Relational Operator4/1 -> Switch/2  "boolean"
  Gain12/1 -> Switch/1
  Switch/1 -> q_t/1
  Saturation/1 -> Sqrt2/1
  Saturation1/1 -> Sqrt4/1
  Sqrt4/1 -> Gain13/1
  Sqrt1/1 -> Gain2/1
  Saturation2/1 -> Sqrt1/1
  Saturation3/1 -> Sqrt3/1
  Sqrt3/1 -> Gain6/1
  Sum10/1 -> Saturation3/1
  [S1] -> Max1/1
  Constant5/1 -> Max1/2
  Max1/1 -> Divide/2
  Max2/1 -> Divide1/2
  Constant6/1 -> Max2/2
  [S1] -> Max2/1
  [S1] -> Max3/1
  Constant7/1 -> Max3/2
  Max3/1 -> Divide2/2
  [S2] -> Max4/1
  Constant8/1 -> Max4/2
  Max4/1 -> Divide3/2
  Max5/1 -> Divide4/2
  Constant9/1 -> Max5/2
  [S2] -> Max5/1
  [S2] -> Max6/1
  Constant10/1 -> Max6/2
  Max6/1 -> Divide5/2
  [S3] -> Max7/1
  Constant11/1 -> Max7/2
  Max7/1 -> Divide6/2
  Constant12/1 -> Max8/2
  [S3] -> Max8/1
  [S3] -> Max9/1
  Constant13/1 -> Max9/2
  Constant14/1 -> Max10/2
  [S4] -> Max10/1
  Max10/1 -> Divide9/2
  [S4] -> Max11/1
  Constant15/1 -> Max11/2
  Max11/1 -> Divide10/2
  Constant16/1 -> Max12/2
  [S4] -> Max12/1
  Max12/1 -> Divide11/2
  Relational Operator5/1 -> Switch1/2
  [tr] -> Relational Operator5/2
  [max] -> Relational Operator5/1
  Constant17/1 -> Switch1/1
  Switch3/1 -> Switch1/3
  Switch1/1 -> Multiport Switch/1  "idx"
  Constant18/1 -> Switch2/1
  Constant19/1 -> Switch2/3
  [max] -> Relational Operator6/1
  [A_22] -> Relational Operator6/2
  Relational Operator6/1 -> Switch2/2
  Relational Operator7/1 -> Switch3/2
  [A_11] -> Relational Operator7/2
  [max] -> Relational Operator7/1
  Constant20/1 -> Switch3/1
  Switch2/1 -> Switch3/3

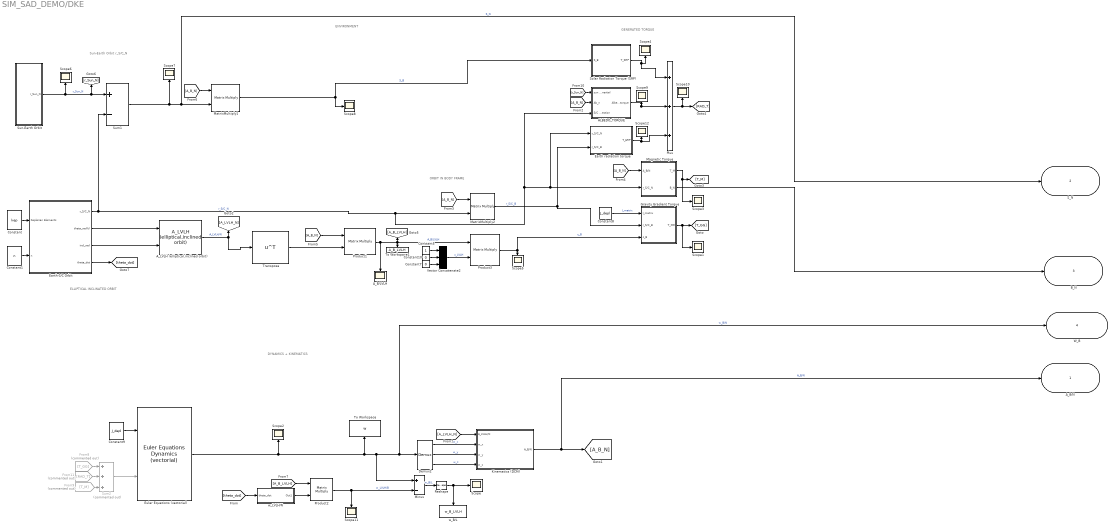
== system SIM_SAD_DEMO/DKE ==
  note: ORBIT IN BODY FRAME
  note: Sun-Earth Orbit r_S/C_N
  note: GENERATED TORQUE
  note: ELLIPTICAL INCLINATED ORBIT
  note: ENVIRONMENT
  note: DYNAMICS + KINEMATICS
  ALBEDO_TORQUE : Subsystem
  A_B/LVLH : Scope
      settings: ActiveDisplayYMinimum=-0.55999388120508109  ActiveDisplayYMaximum=1.1733326534672313
  A_LVLH (elliptical,inclined orbit) : LIBRARY_SAD/A_LVLH (elliptical,inclined orbit)  SystemSampleTime=-1  VariantActivationTime=update diagram  EmptyChoice=off  PassThrough=off  PassThroughVariantControl=(default)  EmptyChoiceVariantControl=(default)  AllowFlexibleInterface=on  Latency=0  AutoFrameSizeCalculation=off
  Constant : Constant  Value=kep
  Constant1 : Constant  Value=n
  Constant10 : Constant  Value=0
  Constant5 : Constant
  Constant7 : Constant  Value=0
  Constant8 : Constant  Value=J_depl
  Constant9 : Constant  Value=J_depl
  Demux2 : Demux  Outputs=3
      settings: DisplayOption=none
  Earth radiation torque : Subsystem
  Earth-S/C Orbit : Subsystem
  Euler Equations (vectorial) : LIBRARY_SAD/Euler Equations Dynamics (vectorial)  SystemSampleTime=-1  VariantActivationTime=update diagram  EmptyChoice=off  PassThrough=off  PassThroughVariantControl=(default)  EmptyChoiceVariantControl=(default)  AllowFlexibleInterface=on  Latency=0  AutoFrameSizeCalculation=off
  From11 : From  Commented=on  GotoTag=RAD_T
  From8 : From  Commented=on  GotoTag=T_GG
  From9 : From  Commented=on  GotoTag=T_M
  Gravity Gradient Torque : Subsystem
  Kinematics (DCM) : Subsystem
  Magnetic Torque : Subsystem
  MatrixMultiply1 : Product  Multiplication=Matrix(*)
  MatrixMultiply2 : Product  Multiplication=Matrix(*)
  Minus : Sum  Inputs=+-
  Plus : Sum  Inputs=+++
  Product1 : Product  Multiplication=Matrix(*)
  Product2 : Product  Multiplication=Matrix(*)
  Product3 : Product  Multiplication=Matrix(*)
  Reshape : Reshape  OutputDimensionality=Customize  OutputDimensions=[3,1]
  Scope{,1..12} (13 alike) : Scope
      Scope settings: ActiveDisplayYMinimum=-0.001958674555984172  ActiveDisplayYMaximum=0.00287841275217951
      Scope1 settings: ActiveDisplayYMinimum=-1  ActiveDisplayYMaximum=1  DataLoggingVariableName=ScopeData3
      Scope10 settings: ActiveDisplayYMinimum=-1  ActiveDisplayYMaximum=1  DataLoggingVariableName=ScopeData27
      Scope11 settings: ActiveDisplayYMinimum=-1  ActiveDisplayYMaximum=1  DataLoggingVariableName=ScopeData21
      Scope12 settings: ActiveDisplayYMinimum=-2.5532417296132574E-10  ActiveDisplayYMaximum=2.6264448663119635E-10  DataLoggingVariableName=ScopeData9
      Scope2 settings: ActiveDisplayYMinimum=-0.00013661573291137518  ActiveDisplayYMaximum=0.0012295415962023768  DataLoggingVariableName=ScopeData2
      Scope3 settings: ActiveDisplayYMinimum=-1  ActiveDisplayYMaximum=1  DataLoggingVariableName=ScopeData4
      Scope4 settings: ActiveDisplayYMinimum=-1  ActiveDisplayYMaximum=1  DataLoggingVariableName=ScopeData16
      Scope5 settings: ActiveDisplayYMinimum=-0.55998948749949928  ActiveDisplayYMaximum=1.1733321652777222  DataLoggingVariableName=ScopeData20
      Scope6 settings: ActiveDisplayYMinimum=-1  ActiveDisplayYMaximum=1  DataLoggingVariableName=ScopeData6
      Scope7 settings: ActiveDisplayYMinimum=-1  ActiveDisplayYMaximum=1  DataLoggingVariableName=ScopeData7
      Scope8 settings: ActiveDisplayYMinimum=-1  ActiveDisplayYMaximum=1  DataLoggingVariableName=ScopeData8
      Scope9 settings: ActiveDisplayYMinimum=-9.2718061255302776E-25  ActiveDisplayYMaximum=9.2718061255302776E-25  DataLoggingVariableName=ScopeData26
  Solar Radiation Torque (SRP) : Subsystem
  Sum1 : Sum  Inputs=+-
  Sum2 : Sum  Commented=on  Inputs=+++
  Sun-Earth Orbit : Subsystem
  To Workspace : ToWorkspace  VariableName=w  SampleTime=-1
  To Workspace1 : ToWorkspace  VariableName=A_B_LVLH  SampleTime=-1
  Transpose : Math  Operator=transpose
  Vector Concatenate2 : Concatenate  NumInputs=3
  w_B/L : ToWorkspace  VariableName=w_B_LVLH  SampleTime=-1
  w_LVLH/N : Subsystem
  A_B/N : Outport
  S_N : Outport  Port=2
  B_N : Outport  Port=3
  W_B : Outport  Port=4
  wires:
  Earth-S/C Orbit/2(theta_rad(t)) -> A_LVLH (elliptical,inclined orbit)/1
  Earth-S/C Orbit/3(incl_rad) -> A_LVLH (elliptical,inclined orbit)/2
  [A_B_N] -> MatrixMultiply2/1
  Sum2/1 -> Euler Equations (vectorial)/2
  [A_B_N] -> ALBEDO_TORQUE/2(Ab_n)
  [A_B_N] -> MatrixMultiply1/1
  Demux2/3 -> Kinematics (DCM)/4(w_z)  "w_z"
  Kinematics (DCM)/1(A_B/N) -> A_B/N/1, [A_B_N]  "A_B/N"
  From9/1 -> Sum2/3
  Earth-S/C Orbit/4(theta_dot) -> [theta_dot]
  A_LVLH (elliptical,inclined orbit)/1 -> Transpose/1, [A_LVLH_N]  "A_LVLH/N"
  Demux2/1 -> Kinematics (DCM)/2(w_x)  "w_x"
  Earth radiation torque/1(T_ERP) -> Plus/3, Scope12/1
  [A_B_N] -> Product1/1
  Solar Radiation Torque (SRP)/1(T_SRP) -> Scope4/1, Plus/1
  MatrixMultiply1/1 -> Scope8/1, Solar Radiation Torque (SRP)/1(S_B)  "S_B"
  Constant7/1 -> Vector Concatenate2/3
  Constant10/1 -> Vector Concatenate2/2
  Constant9/1 -> Euler Equations (vectorial)/1
  [A_LVLH_N] -> Kinematics (DCM)/1(A_LVLH/N)
  Constant8/1 -> Gravity Gradient Torque/1(I_matrix)  "I_matrix"
  Sum1/1 -> S_N/1, MatrixMultiply1/2, Scope7/1  "S_N"
  From11/1 -> Sum2/2
  Constant/1 -> Earth-S/C Orbit/1(Keplerian Elements)
  Constant1/1 -> Earth-S/C Orbit/2(n)
  [A_B_LVLH] -> Product2/1
  [r_Sun_N] -> ALBEDO_TORQUE/1(sun direction inertial)
  Product1/1 -> Product3/1, [A_B_LVLH], To Workspace1/1, A_B/LVLH/1  "A_B/LVLH"
  Transpose/1 -> Product1/2
  Product2/1 -> Minus/2, Scope11/1  "w_LVLH/B"
  Minus/1 -> Reshape/1  "w_B/L"
  w_LVLH/N/1(Out1) -> Product2/2
  Reshape/1 -> Scope/1, w_B/L/1
  ALBEDO_TORQUE/1(Albedo_torque) -> Scope9/1, Plus/2
  From8/1 -> Sum2/1
  [A_B_N] -> Magnetic Torque/1(A_B/N)
  Earth-S/C Orbit/1(r_S/C_N) -> Sum1/2, ALBEDO_TORQUE/3(S/C direction), Magnetic Torque/2(r_S/C_N), Earth radiation torque/1(r_S/C_N), MatrixMultiply2/2  "r_S/C_N"
  Plus/1 -> [RAD_T], Scope10/1
  Euler Equations (vectorial)/1 -> W_B/1, Demux2/1, Minus/1, To Workspace/1, Scope2/1  "w_B/N"
  Product3/1 -> Gravity Gradient Torque/3(c_B), Scope5/1  "c_B"
  Demux2/2 -> Kinematics (DCM)/3(w_y)  "w_y"
  Constant5/1 -> Vector Concatenate2/1
  Gravity Gradient Torque/1(T_GG) -> Scope1/1, [T_GG]
  MatrixMultiply2/1 -> Gravity Gradient Torque/2(r_S/C_B), Earth radiation torque/2(r_S/C_B)  "r_S/C_B"
  [theta_dot] -> w_LVLH/N/1(theta_dot)
  Magnetic Torque/1(T_M) -> Scope3/1, [T_M]
  Vector Concatenate2/1 -> Product3/2  "c_LVLH"
  Magnetic Torque/2(B_N) -> B_N/1
  Sun-Earth Orbit/1(r_Sun_N) -> Sum1/1, [r_Sun_N], Scope6/1  "r_Sun_N"

== system SIM_SAD_DEMO/SENSORS ==
  A_B/N : Inport
  S_N : Inport  Port=2
  "B_N " : Inport  Port=3
  w_B : Inport  Port=4
  Discrete Transfer Fcn1 : DiscreteTransferFcn  LoadFcn=dspblkCoreblockFVToolHelper(gcbh,'load');  Numerator=bvec  Denominator=avec
      settings: CopyFcn=dspblkCoreblockFVToolHelper(gcbh,'copy');  DeleteFcn=dspblkCoreblockFVToolHelper(gcbh,'close');  ModelCloseFcn=dspblkCoreblockFVToolHelper(gcbh,'close');  PreSaveFcn=dspblkCoreblockFVToolHelper(gcbh,'presave');  PostSaveFcn=dspblkCoreblockFVToolHelper(gcbh,'postsave');  CloseFcn=dspblkCoreblockFVToolHelper(gcbh,'close');
  Discrete Transfer Fcn2 : DiscreteTransferFcn  LoadFcn=dspblkCoreblockFVToolHelper(gcbh,'load');  Numerator=bvec  Denominator=avec
      settings: CopyFcn=dspblkCoreblockFVToolHelper(gcbh,'copy');  DeleteFcn=dspblkCoreblockFVToolHelper(gcbh,'close');  ModelCloseFcn=dspblkCoreblockFVToolHelper(gcbh,'close');  PreSaveFcn=dspblkCoreblockFVToolHelper(gcbh,'presave');  PostSaveFcn=dspblkCoreblockFVToolHelper(gcbh,'postsave');  CloseFcn=dspblkCoreblockFVToolHelper(gcbh,'close');
  Divide : Product  Inputs=*/
  Divide1 : Product  Inputs=*/
  Divide2 : Product  Inputs=*/
  Gyroscope : Subsystem
  Magnetometer : Subsystem
  Sun Sensor : Subsystem
  vector_norm : LIBRARY_SAD/vector_norm  SystemSampleTime=-1  VariantActivationTime=update diagram  EmptyChoice=off  PassThrough=off  PassThroughVariantControl=(default)  EmptyChoiceVariantControl=(default)  AllowFlexibleInterface=on  Latency=0  AutoFrameSizeCalculation=off
  vector_norm1 : LIBRARY_SAD/vector_norm  SystemSampleTime=-1  VariantActivationTime=update diagram  EmptyChoice=off  PassThrough=off  PassThroughVariantControl=(default)  EmptyChoiceVariantControl=(default)  AllowFlexibleInterface=on  Latency=0  AutoFrameSizeCalculation=off
  vector_norm2 : LIBRARY_SAD/vector_norm  SystemSampleTime=-1  VariantActivationTime=update diagram  EmptyChoice=off  PassThrough=off  PassThroughVariantControl=(default)  EmptyChoiceVariantControl=(default)  AllowFlexibleInterface=on  Latency=0  AutoFrameSizeCalculation=off
  s1_B : Outport
  s2_B : Outport  Port=2
  w_B_m : Outport  Port=3
  wires:
  A_B/N/1 -> Sun Sensor/1(A_B/N), Magnetometer/2(A_B/N)
  S_N/1 -> vector_norm/1, Divide/1
  Divide/1 -> Sun Sensor/2(v1_N)  "S_N_hat"
  vector_norm/1 -> Divide/2
  "B_N "/1 -> Magnetometer/1(v2_N)
  Magnetometer/1(s2_B) -> Discrete Transfer Fcn1/1
  vector_norm1/1 -> Divide1/2
  Divide1/1 -> s2_B/1
  Sun Sensor/1(s1_B) -> Discrete Transfer Fcn2/1
  vector_norm2/1 -> Divide2/2
  Divide2/1 -> s1_B/1
  Gyroscope/1(w_m) -> w_B_m/1
  w_B/1 -> Gyroscope/1(w_B (rad/s))
  Discrete Transfer Fcn1/1 -> Divide1/1, vector_norm1/1
  Discrete Transfer Fcn2/1 -> Divide2/1, vector_norm2/1

== system SIM_SAD_DEMO/STATE-SPACE MODEL ==
  w_est : Inport
  A_B/T_e : Inport  Port=2
  Demux : Demux  Outputs=9
  Display : Display
  Display1 : Display
  Display2 : Display
  Gain : Gain  Gain=0.5
  Gain1 : Gain  Gain=0.5
  Gain2 : Gain  Gain=0.5
  Reshape : Reshape  OutputDimensionality=Customize  OutputDimensions=[9,1]
  Sum : Sum  Inputs=+-
  Sum1 : Sum  Inputs=+-
  Sum2 : Sum  Inputs=+-
  Terminator : Terminator
  Terminator1 : Terminator
  Terminator2 : Terminator
  Vector Concatenate : Concatenate  NumInputs=3
  Vector Concatenate1 : Concatenate
  x : Outport
  wires:
  A_B/T_e/1 -> Reshape/1
  Reshape/1 -> Demux/1
  Demux/1 -> Terminator1/1  "A_11"
  Demux/2 -> Sum2/2  "A_21"
  Demux/3 -> Sum1/1  "A_31"
  Demux/4 -> Sum2/1  "A_12"
  Demux/5 -> Terminator/1  "A_22"
  Demux/6 -> Sum/2  "A_32"
  Demux/7 -> Sum1/2  "A_13"
  Demux/8 -> Sum/1  "A_23"
  Demux/9 -> Terminator2/1  "A_33"
  Sum/1 -> Gain/1
  Sum1/1 -> Gain1/1
  Sum2/1 -> Gain2/1
  Gain/1 -> Vector Concatenate/1  "x1"
  Gain1/1 -> Vector Concatenate/2  "x2"
  Gain2/1 -> Vector Concatenate/3  "x3"
  Vector Concatenate/1 -> Vector Concatenate1/1, Display/1
  w_est/1 -> Vector Concatenate1/2, Display1/1  "x4,x5,x6"
  Vector Concatenate1/1 -> x/1, Display2/1  "x"

== system SIM_SAD_DEMO/q-->DCM ==
  note: ORTHONORMALITY ERROR A_B/N RECONSTRUCTED CHECK
  q_e : Inport
  Demux1 : Demux  Outputs=9
  Demux2 : Demux
  Display : Display
  Gain4 : Gain  Gain=2
  Gain5 : Gain  Gain=2
  I : Constant  Value=[1,0,0;0,1,0;0,0,1]
  I1 : Constant  Value=[1,0,0;0,1,0;0,0,1]
  MatrixMultiply : Product  Multiplication=Matrix(*)
  MatrixMultiply1 : Product  Multiplication=Matrix(*)
  MatrixMultiply2 : Product  Multiplication=Matrix(*)
  Product1 : Product
  Product2 : Product
  Reshape1 : Reshape  OutputDimensionality=Customize  OutputDimensions=[9,1]
  Scope : Scope
      settings: ActiveDisplayYMinimum=-1  ActiveDisplayYMaximum=1  DataLoggingVariableName=ScopeData57
  Scope1 : Scope  NumInputPorts=9
      settings: ActiveDisplayYMinimum=0.78091180257448345  ActiveDisplayYMaximum=1.0243231881597876  DataLoggingVariableName=ScopeData56
  Square : Math  Operator=square
  Sum4 : Sum  Inputs=+-
  Sum5 : Sum  Inputs=+-
  Sum6 : Sum  Inputs=-++
  Transpose : Math  Operator=transpose
  Transpose2 : Math  Operator=transpose
  Vector Concatenate1 : Concatenate  NumInputs=3
  "[qΛ]" : Subsystem
  A_B/N_e : Outport
  wires:
  Demux1/2 -> Scope1/2  "A_12"
  MatrixMultiply/1 -> Sum4/2  "qTq"
  Demux2/3 -> Vector Concatenate1/3
  Gain5/1 -> Product1/2  "2q4"
  Product1/1 -> Sum6/1  "2*q4*[qΛ ]"
  Demux2/4 -> Gain5/1, Square/1  "q4"
  Demux1/6 -> Scope1/6  "A_23"
  Product2/1 -> Sum6/2  "(q4^2-qTq)*I"
  Demux2/1 -> Vector Concatenate1/1
  Gain4/1 -> Sum6/3  "2*q*qT"
  Demux1/5 -> Scope1/5  "A_22"
  I1/1 -> Sum5/2
  "[qΛ]"/1("[qΛ]") -> Product1/1
  MatrixMultiply1/1 -> Gain4/1  "qqT"
  Transpose2/1 -> MatrixMultiply2/1  "qT"
  Square/1 -> Sum4/1
  Demux1/8 -> Scope1/8  "A_32"
  Sum4/1 -> Product2/1
  Demux1/7 -> Scope1/7  "A_31"
  I/1 -> Product2/2
  Sum5/1 -> Scope/1
  Demux1/9 -> Scope1/9  "A_33"
  Vector Concatenate1/1 -> Transpose/1, MatrixMultiply1/1, MatrixMultiply/2  "q"
  Demux2/2 -> Vector Concatenate1/2
  Sum6/1 -> Transpose2/1, MatrixMultiply2/2, Reshape1/1, A_B/N_e/1  "A_B/N"
  Demux1/1 -> Scope1/1  "A_11"
  MatrixMultiply2/1 -> Sum5/1  "qTq"
  Demux1/4 -> Scope1/4  "A_21"
  Transpose/1 -> MatrixMultiply1/2, MatrixMultiply/1  "qT"
  Reshape1/1 -> Demux1/1
  q_e/1 -> Demux2/1, "[qΛ]"/1(q), Display/1
  Demux1/3 -> Scope1/3  "A_13"

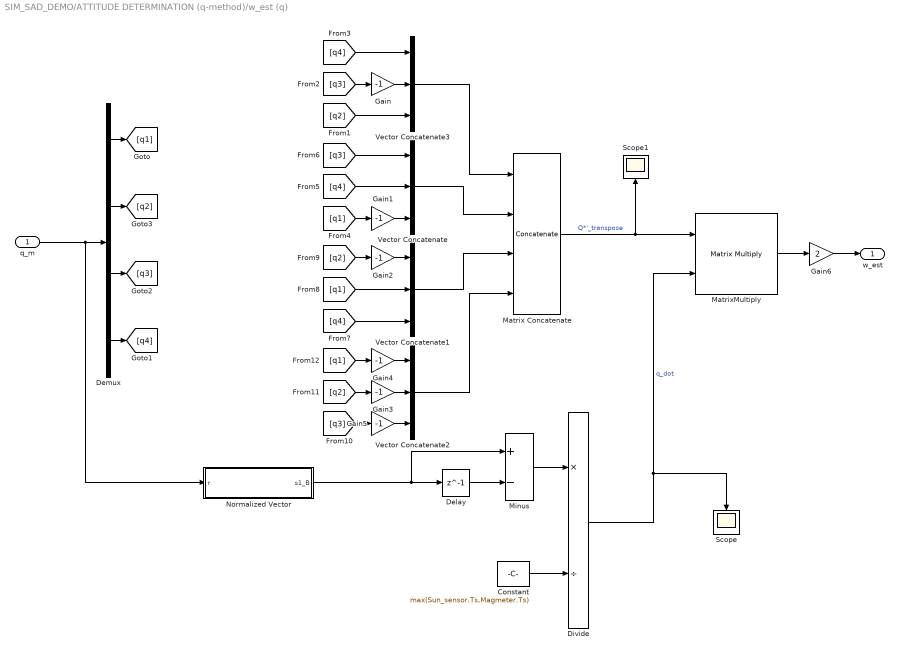
== system SIM_SAD_DEMO/ATTITUDE DETERMINATION (q-method)/w_est (q) ==
  q_m : Inport
  Constant : Constant  Value=max(Sun_sensor.Ts,Magmeter.Ts)
  Delay : Delay  DelayLength=1
  Demux : Demux
  Divide : Product  Inputs=*/
  Gain{,1..5} (6 alike) : Gain  Gain=-1
  Gain6 : Gain  Gain=2
  Matrix Concatenate : Concatenate  NumInputs=4  Mode=Multidimensional array  ConcatenateDimension=2
  MatrixMultiply : Product  Multiplication=Matrix(*)
  Minus : Sum  Inputs=+-
  Normalized Vector : Subsystem
  Scope : Scope
      settings: ActiveDisplayYMinimum=-1  ActiveDisplayYMaximum=1  DataLoggingVariableName=ScopeData67
  Scope1 : Scope
      settings: ActiveDisplayYMinimum=-1  ActiveDisplayYMaximum=1  DataLoggingVariableName=ScopeData68
  Vector Concatenate{,1..3} (4 alike) : Concatenate  NumInputs=3
  w_est : Outport
  wires:
  q_m/1 -> Normalized Vector/1(r), Demux/1
  Demux/1 -> [q1]
  Demux/2 -> [q2]
  Demux/3 -> [q3]
  Demux/4 -> [q4]
  [q4] -> Vector Concatenate3/1
  [q3] -> Gain/1
  Gain/1 -> Vector Concatenate3/2
  [q2] -> Vector Concatenate3/3
  [q1] -> Gain1/1
  [q3] -> Vector Concatenate/1
  [q4] -> Vector Concatenate1/3
  [q2] -> Gain2/1
  [q3] -> Gain5/1
  [q2] -> Gain3/1
  [q1] -> Gain4/1
  Gain3/1 -> Vector Concatenate2/2
  [q1] -> Vector Concatenate1/2
  [q4] -> Vector Concatenate/2
  Gain1/1 -> Vector Concatenate/3
  Gain2/1 -> Vector Concatenate1/1
  Gain4/1 -> Vector Concatenate2/1
  Gain5/1 -> Vector Concatenate2/3
  Vector Concatenate3/1 -> Matrix Concatenate/1
  Vector Concatenate/1 -> Matrix Concatenate/2
  Vector Concatenate1/1 -> Matrix Concatenate/3
  Vector Concatenate2/1 -> Matrix Concatenate/4
  Delay/1 -> Minus/2
  Matrix Concatenate/1 -> MatrixMultiply/1, Scope1/1  "Q*'_transpose"
  MatrixMultiply/1 -> Gain6/1
  Gain6/1 -> w_est/1
  Minus/1 -> Divide/1
  Divide/1 -> Scope/1, MatrixMultiply/2  "q_dot"
  Constant/1 -> Divide/2
  Normalized Vector/1(s1_B) -> Delay/1, Minus/1

== system SIM_SAD_DEMO/ATTITUDE TARGET (Sun Pointing)/Normalized Vector ==
  In1 : Inport
  Divide : Product  Inputs=*/
  vector_norm : LIBRARY_SAD/vector_norm  SystemSampleTime=-1  VariantActivationTime=update diagram  EmptyChoice=off  PassThrough=off  PassThroughVariantControl=(default)  EmptyChoiceVariantControl=(default)  AllowFlexibleInterface=on  Latency=0  AutoFrameSizeCalculation=off
  Out1 : Outport
  wires:
  vector_norm/1 -> Divide/2
  In1/1 -> Divide/1, vector_norm/1
  Divide/1 -> Out1/1

== system SIM_SAD_DEMO/ATTITUDE TARGET (Sun Pointing)/Normalized Vector2 ==
  r : Inport
  Divide : Product  Inputs=*/
  vector_norm : LIBRARY_SAD/vector_norm  SystemSampleTime=-1  VariantActivationTime=update diagram  EmptyChoice=off  PassThrough=off  PassThroughVariantControl=(default)  EmptyChoiceVariantControl=(default)  AllowFlexibleInterface=on  Latency=0  AutoFrameSizeCalculation=off
  s2_B : Outport
  wires:
  Divide/1 -> s2_B/1
  r/1 -> Divide/1, vector_norm/1
  vector_norm/1 -> Divide/2

== system SIM_SAD_DEMO/DCM ---> q/q-->DCM (CHECK) ==
  note: ORTHONORMALITY ERROR A_B/N RECONSTRUCTED CHECK
  q_norm : Inport
  Demux1 : Demux  Outputs=9
  Demux2 : Demux
  Display : Display
  Gain4 : Gain  Gain=2
  Gain5 : Gain  Gain=2
  I : Constant  Value=[1,0,0;0,1,0;0,0,1]
  I1 : Constant  Value=[1,0,0;0,1,0;0,0,1]
  MatrixMultiply : Product  Multiplication=Matrix(*)
  MatrixMultiply1 : Product  Multiplication=Matrix(*)
  MatrixMultiply2 : Product  Multiplication=Matrix(*)
  Product1 : Product
  Product2 : Product
  Reshape1 : Reshape  OutputDimensionality=Customize  OutputDimensions=[9,1]
  Scope : Scope
      settings: ActiveDisplayYMinimum=-1  ActiveDisplayYMaximum=1  DataLoggingVariableName=ScopeData57
  Scope1 : Scope  NumInputPorts=9
      settings: ActiveDisplayYMinimum=-1.2499999988864972  ActiveDisplayYMaximum=1.2499999998762776  DataLoggingVariableName=ScopeData56
  Square : Math  Operator=square
  Sum4 : Sum  Inputs=+-
  Sum5 : Sum  Inputs=+-
  Sum6 : Sum  Inputs=-++
  Transpose : Math  Operator=transpose
  Transpose2 : Math  Operator=transpose
  Vector Concatenate1 : Concatenate  NumInputs=3
  "[qΛ]" : Subsystem
  wires:
  Demux1/3 -> Scope1/3  "A_13"
  q_norm/1 -> Display/1, "[qΛ]"/1(q), Demux2/1
  Reshape1/1 -> Demux1/1
  Transpose/1 -> MatrixMultiply/1, MatrixMultiply1/2  "qT"
  Demux1/4 -> Scope1/4  "A_21"
  MatrixMultiply2/1 -> Sum5/1  "qTq"
  Demux1/1 -> Scope1/1  "A_11"
  Sum6/1 -> Reshape1/1, MatrixMultiply2/2, Transpose2/1  "A_B/N"
  Demux2/2 -> Vector Concatenate1/2
  Vector Concatenate1/1 -> MatrixMultiply/2, MatrixMultiply1/1, Transpose/1  "q"
  Demux1/9 -> Scope1/9  "A_33"
  Sum5/1 -> Scope/1
  I/1 -> Product2/2
  Demux1/7 -> Scope1/7  "A_31"
  Sum4/1 -> Product2/1
  Demux1/8 -> Scope1/8  "A_32"
  Square/1 -> Sum4/1
  Transpose2/1 -> MatrixMultiply2/1  "qT"
  MatrixMultiply1/1 -> Gain4/1  "qqT"
  "[qΛ]"/1("[qΛ]") -> Product1/1
  I1/1 -> Sum5/2
  Demux1/5 -> Scope1/5  "A_22"
  Gain4/1 -> Sum6/3  "2*q*qT"
  Demux2/1 -> Vector Concatenate1/1
  Product2/1 -> Sum6/2  "(q4^2-qTq)*I"
  Demux1/6 -> Scope1/6  "A_23"
  Demux2/4 -> Square/1, Gain5/1  "q4"
  Product1/1 -> Sum6/1  "2*q4*[qΛ ]"
  Gain5/1 -> Product1/2  "2q4"
  Demux2/3 -> Vector Concatenate1/3
  MatrixMultiply/1 -> Sum4/2  "qTq"
  Demux1/2 -> Scope1/2  "A_12"

== system SIM_SAD_DEMO/DCM ---> q/vector_norm ==
  r : Inport
  Sqrt : Sqrt
  Square : Math  Operator=square
  Sum of Elements : Sum  Inputs=+
  r_norm : Outport
  wires:
  Sqrt/1 -> r_norm/1
  r/1 -> Square/1
  Sum of Elements/1 -> Sqrt/1
  Square/1 -> Sum of Elements/1
